simulink model "Copy_of_AB_Final_of_MPC_Bandwidth_Result"  (R2022b)
settings: Solver=FixedStepDiscrete  StartTime=0.0  StopTime=Inf  FixedStep=100e-6  RelTol=1e-3  EnableMultiTasking=on
undefined symbols (not defined in the file): C28x, CPU1, CPU2, CurrentBypassValue, DiscIntNeverNeededParam, Down, GPTRIP1SEL, TZ1, Up
libraries: c2802xlib x31, simulink x22, dspstat3 x17, dspsigops x9, c2837xDlib x6, c280xlib x5, PID_Lib x2, c2000lib x1, spsAlphaBetaZerotoabcLib x1, spsAlphaBetaZerotodq0Lib x1
(part 8 of 8)

== system Copy_of_AB_Final_of_MPC_Bandwidth_Result/Subsystem1/GridCurrentSecondPrediction/CostFunctionofVoltageVectors/CostFunctionVoltage3/QGridCurrentSecondPrediction_Voltage3 ==
  MPCC_f32Predictionterm_A : Inport
  MPCC_f32Predictionterm_B : Inport  Port=2
  MPCC_f32Predictionterm_C : Inport  Port=3
  MPCC_f32DGridCurrent_K_1 : Inport  Port=4
  MPCC_f32QGridCurrent_K_1 : Inport  Port=5
  MPCC_f32QGridVoltage : Inport  Port=6
  MPCC_f32QVoltageVector3 : Inport  Port=7
  Add1 : Sum  Inputs=+-+-
  Gain : Gain  Gain=0
  Product : Product
  Product1 : Product
  Product2 : Product  OutDataTypeStr=Inherit: Inherit via back propagation
  Product4 : Product
  MPCC_f32QGridCurrent_K_2_Voltage3 : Outport
  wires:
  [MPCC_f32QGridCurrent_K_1] -> Product/2
  MPCC_f32Predictionterm_A/1 -> [MPCC_f32Predictionterm_A]
  [MPCC_f32QGridVoltage] -> Product2/2
  Product1/1 -> Gain/1
  [MPCC_f32Predictionterm_C] -> Product1/1
  Product/1 -> Add1/1
  [MPCC_f32QVoltageVector3] -> Product4/2
  [MPCC_f32Predictionterm_A] -> Product/1
  [MPCC_f32Predictionterm_B] -> Product4/1
  [MPCC_f32Predictionterm_B] -> Product2/1
  [MPCC_f32DGridCurrent_K_1] -> Product1/2
  MPCC_f32DGridCurrent_K_1/1 -> [MPCC_f32DGridCurrent_K_1]
  MPCC_f32QGridCurrent_K_1/1 -> [MPCC_f32QGridCurrent_K_1]
  MPCC_f32Predictionterm_C/1 -> [MPCC_f32Predictionterm_C]
  MPCC_f32QGridVoltage/1 -> [MPCC_f32QGridVoltage]
  MPCC_f32Predictionterm_B/1 -> [MPCC_f32Predictionterm_B]
  Add1/1 -> MPCC_f32QGridCurrent_K_2_Voltage3/1
  MPCC_f32QVoltageVector3/1 -> [MPCC_f32QVoltageVector3]
  Product2/1 -> Add1/3
  Product4/1 -> Add1/4
  Gain/1 -> Add1/2

== system Copy_of_AB_Final_of_MPC_Bandwidth_Result/Subsystem1/GridCurrentSecondPrediction/CostFunctionofVoltageVectors/CostFunctionVoltage4/CostFunctionVoltage4 ==
  MPCC_f32DGridCurrentReference : Inport
  MPCC_f32QGridCurrentReference : Inport  Port=2
  MPCC_f32DGridCurrent_K_2_Voltage4 : Inport  Port=3
  MPCC_f32QGridCurrent_K_2_Voltage4 : Inport  Port=4
  MPCC_f32DGridCurrent : Inport  Port=5
  MPCC_f32QGridCurrent : Inport  Port=6
  MPCC_f32DGridCurrent1 : Inport  Port=7
  MPCC_f32QGridCurrent1 : Inport  Port=8
  Abs{,1..5} (6 alike) : Abs  SaturateOnIntegerOverflow=off
  Add{,2..6} (6 alike) : Sum  Inputs=+-
  Add1 : Sum  Inputs=++++++
  Constant : Constant  Value=single(0)
  Constant1 : Constant  Value=single(0)
  Gain : Gain
  Gain1 : Gain
  Gain2 : Gain  Gain=0
  Gain3 : Gain  Gain=0
  Square : Math  Operator=square
  Square1 : Math  Operator=square
  MPCC_f32CostFunction_Voltage4 : Outport
  wires:
  MPCC_f32QGridCurrentReference/1 -> [MPCC_f32QGridCurrentReference]
  MPCC_f32DGridCurrentReference/1 -> [MPCC_f32DGridCurrentReference]
  MPCC_f32QGridCurrent_K_2_Voltage4/1 -> [MPCC_f32QGridCurrent_K_2_Voltage4]
  MPCC_f32DGridCurrent_K_2_Voltage4/1 -> [MPCC_f32DGridCurrent_K_2_Voltage4]
  [MPCC_f32DGridCurrentReference] -> Add/1
  [MPCC_f32DGridCurrent_K_2_Voltage4] -> Add/2
  [MPCC_f32QGridCurrentReference] -> Add2/1
  [MPCC_f32QGridCurrent_K_2_Voltage4] -> Add2/2
  MPCC_f32QGridCurrent/1 -> [MPCC_f32QGridCurrent]
  MPCC_f32DGridCurrent/1 -> [MPCC_f32DGridCurrent]
  [MPCC_f32QGridCurrent] -> Add4/1
  Add4/1 -> Abs3/1
  Add3/1 -> Abs2/1
  [MPCC_f32QGridCurrent_K_2_Voltage4] -> Add4/2
  [MPCC_f32DGridCurrent] -> Add3/1
  [MPCC_f32DGridCurrent_K_2_Voltage4] -> Add3/2
  Abs2/1 -> Gain/1
  Abs3/1 -> Gain1/1
  Add1/1 -> MPCC_f32CostFunction_Voltage4/1
  Gain/1 -> Add1/3
  Gain1/1 -> Add1/4
  Abs1/1 -> Add1/2
  Add2/1 -> Abs1/1
  Abs/1 -> Add1/1
  Add/1 -> Abs/1
  MPCC_f32DGridCurrent1/1 -> [MPCC_f32DGridCurrent1]
  MPCC_f32QGridCurrent1/1 -> [MPCC_f32QGridCurrent1]
  Constant/1 -> Add5/1
  Add5/1 -> Abs4/1
  Add6/1 -> Abs5/1
  Abs4/1 -> Gain2/1
  Constant1/1 -> Add6/1
  [MPCC_f32DGridCurrent1] -> Add6/2
  [MPCC_f32QGridCurrent1] -> Add5/2
  Gain2/1 -> Add1/6
  Abs5/1 -> Gain3/1
  Gain3/1 -> Add1/5

== system Copy_of_AB_Final_of_MPC_Bandwidth_Result/Subsystem1/GridCurrentSecondPrediction/CostFunctionofVoltageVectors/CostFunctionVoltage4/DGridCurrentSecondPrediction_Voltage4 ==
  MPCC_f32Predictionterm_A : Inport
  MPCC_f32Predictionterm_B : Inport  Port=2
  MPCC_f32Predictionterm_C : Inport  Port=3
  MPCC_f32DGridCurrent_K_1 : Inport  Port=4
  MPCC_f32QGridCurrent_K_1 : Inport  Port=5
  MPCC_f32DGridVoltage : Inport  Port=6
  MPCC_f32DVoltageVector4 : Inport  Port=7
  Add1 : Sum  Inputs=+++-
  Gain : Gain  Gain=0
  Product : Product
  Product1 : Product
  Product2 : Product  OutDataTypeStr=Inherit: Inherit via back propagation
  Product4 : Product
  MPCC_f32DGridCurrent_K_2_Voltage4 : Outport
  wires:
  [MPCC_f32DGridCurrent_K_1] -> Product/2
  MPCC_f32Predictionterm_A/1 -> [MPCC_f32Predictionterm_A]
  [MPCC_f32DGridVoltage] -> Product2/2
  Product1/1 -> Gain/1
  [MPCC_f32Predictionterm_C] -> Product1/1
  Product/1 -> Add1/1
  [MPCC_f32DVoltageVector4] -> Product4/2
  MPCC_f32DGridVoltage/1 -> [MPCC_f32DGridVoltage]
  [MPCC_f32Predictionterm_A] -> Product/1
  [MPCC_f32Predictionterm_B] -> Product4/1
  [MPCC_f32Predictionterm_B] -> Product2/1
  [MPCC_f32QGridCurrent_K_1] -> Product1/2
  MPCC_f32DGridCurrent_K_1/1 -> [MPCC_f32DGridCurrent_K_1]
  MPCC_f32QGridCurrent_K_1/1 -> [MPCC_f32QGridCurrent_K_1]
  MPCC_f32Predictionterm_C/1 -> [MPCC_f32Predictionterm_C]
  MPCC_f32Predictionterm_B/1 -> [MPCC_f32Predictionterm_B]
  Add1/1 -> MPCC_f32DGridCurrent_K_2_Voltage4/1
  MPCC_f32DVoltageVector4/1 -> [MPCC_f32DVoltageVector4]
  Product2/1 -> Add1/3
  Product4/1 -> Add1/4
  Gain/1 -> Add1/2

== system Copy_of_AB_Final_of_MPC_Bandwidth_Result/Subsystem1/GridCurrentSecondPrediction/CostFunctionofVoltageVectors/CostFunctionVoltage4/QGridCurrentSecondPrediction_Voltage4 ==
  MPCC_f32Predictionterm_A : Inport
  MPCC_f32Predictionterm_B : Inport  Port=2
  MPCC_f32Predictionterm_C : Inport  Port=3
  MPCC_f32DGridCurrent_K_1 : Inport  Port=4
  MPCC_f32QGridCurrent_K_1 : Inport  Port=5
  MPCC_f32QGridVoltage : Inport  Port=6
  MPCC_f32QVoltageVector4 : Inport  Port=7
  Add1 : Sum  Inputs=+-+-
  Gain : Gain  Gain=0
  Product : Product
  Product1 : Product
  Product2 : Product  OutDataTypeStr=Inherit: Inherit via back propagation
  Product4 : Product  OutDataTypeStr=Inherit: Inherit via back propagation
  MPCC_f32QGridCurrent_K_2_Voltage4 : Outport
  wires:
  [MPCC_f32QGridCurrent_K_1] -> Product/2
  MPCC_f32Predictionterm_A/1 -> [MPCC_f32Predictionterm_A]
  [MPCC_f32QGridVoltage] -> Product2/2
  Product1/1 -> Gain/1
  [MPCC_f32Predictionterm_C] -> Product1/1
  Product/1 -> Add1/1
  [MPCC_f32QVoltageVector4] -> Product4/2
  [MPCC_f32Predictionterm_A] -> Product/1
  [MPCC_f32Predictionterm_B] -> Product4/1
  [MPCC_f32Predictionterm_B] -> Product2/1
  [MPCC_f32DGridCurrent_K_1] -> Product1/2
  MPCC_f32DGridCurrent_K_1/1 -> [MPCC_f32DGridCurrent_K_1]
  MPCC_f32QGridCurrent_K_1/1 -> [MPCC_f32QGridCurrent_K_1]
  MPCC_f32Predictionterm_C/1 -> [MPCC_f32Predictionterm_C]
  MPCC_f32QGridVoltage/1 -> [MPCC_f32QGridVoltage]
  MPCC_f32Predictionterm_B/1 -> [MPCC_f32Predictionterm_B]
  Add1/1 -> MPCC_f32QGridCurrent_K_2_Voltage4/1
  MPCC_f32QVoltageVector4/1 -> [MPCC_f32QVoltageVector4]
  Product2/1 -> Add1/3
  Product4/1 -> Add1/4
  Gain/1 -> Add1/2

== system Copy_of_AB_Final_of_MPC_Bandwidth_Result/Subsystem1/GridCurrentSecondPrediction/CostFunctionofVoltageVectors/CostFunctionVoltage5/CostFunctionVoltage5 ==
  MPCC_f32DGridCurrentReference : Inport
  MPCC_f32QGridCurrentReference : Inport  Port=2
  MPCC_f32DGridCurrent_K_2_Voltage5 : Inport  Port=3
  MPCC_f32QGridCurrent_K_2_Voltage5 : Inport  Port=4
  MPCC_f32DGridCurrent : Inport  Port=5
  MPCC_f32QGridCurrent : Inport  Port=6
  MPCC_f32DGridCurrent1 : Inport  Port=7
  MPCC_f32QGridCurrent1 : Inport  Port=8
  Abs{,1..5} (6 alike) : Abs  SaturateOnIntegerOverflow=off
  Add{,2..6} (6 alike) : Sum  Inputs=+-
  Add1 : Sum  Inputs=++++++
  Constant : Constant  Value=single(0)
  Constant1 : Constant  Value=single(0)
  Gain : Gain
  Gain1 : Gain
  Gain2 : Gain  Gain=0
  Gain3 : Gain  Gain=0
  Square : Math  Operator=square
  Square1 : Math  Operator=square
  MPCC_f32CostFunction_Voltage5 : Outport
  wires:
  MPCC_f32QGridCurrentReference/1 -> [MPCC_f32QGridCurrentReference]
  MPCC_f32DGridCurrentReference/1 -> [MPCC_f32DGridCurrentReference]
  MPCC_f32QGridCurrent_K_2_Voltage5/1 -> [MPCC_f32QGridCurrent_K_2_Voltage5]
  MPCC_f32DGridCurrent_K_2_Voltage5/1 -> [MPCC_f32DGridCurrent_K_2_Voltage5]
  [MPCC_f32DGridCurrentReference] -> Add/1
  [MPCC_f32DGridCurrent_K_2_Voltage5] -> Add/2
  [MPCC_f32QGridCurrentReference] -> Add2/1
  [MPCC_f32QGridCurrent_K_2_Voltage5] -> Add2/2
  MPCC_f32QGridCurrent/1 -> [MPCC_f32QGridCurrent]
  MPCC_f32DGridCurrent/1 -> [MPCC_f32DGridCurrent]
  [MPCC_f32QGridCurrent] -> Add4/1
  Add4/1 -> Abs3/1
  Add3/1 -> Abs2/1
  [MPCC_f32QGridCurrent_K_2_Voltage5] -> Add4/2
  [MPCC_f32DGridCurrent] -> Add3/1
  [MPCC_f32DGridCurrent_K_2_Voltage5] -> Add3/2
  Abs2/1 -> Gain/1
  Abs3/1 -> Gain1/1
  Add1/1 -> MPCC_f32CostFunction_Voltage5/1
  Gain/1 -> Add1/3
  Gain1/1 -> Add1/4
  Abs1/1 -> Add1/2
  Add2/1 -> Abs1/1
  Abs/1 -> Add1/1
  Add/1 -> Abs/1
  MPCC_f32DGridCurrent1/1 -> [MPCC_f32DGridCurrent1]
  MPCC_f32QGridCurrent1/1 -> [MPCC_f32QGridCurrent1]
  Constant/1 -> Add5/1
  Add5/1 -> Abs4/1
  Add6/1 -> Abs5/1
  Abs4/1 -> Gain2/1
  Constant1/1 -> Add6/1
  [MPCC_f32DGridCurrent1] -> Add6/2
  [MPCC_f32QGridCurrent1] -> Add5/2
  Gain2/1 -> Add1/6
  Abs5/1 -> Gain3/1
  Gain3/1 -> Add1/5

== system Copy_of_AB_Final_of_MPC_Bandwidth_Result/Subsystem1/GridCurrentSecondPrediction/CostFunctionofVoltageVectors/CostFunctionVoltage5/DGridCurrentSecondPrediction_Voltage5 ==
  MPCC_f32Predictionterm_A : Inport
  MPCC_f32Predictionterm_B : Inport  Port=2
  MPCC_f32Predictionterm_C : Inport  Port=3
  MPCC_f32DGridCurrent_K_1 : Inport  Port=4
  MPCC_f32QGridCurrent_K_1 : Inport  Port=5
  MPCC_f32DGridVoltage : Inport  Port=6
  MPCC_f32DVoltageVector5 : Inport  Port=7
  Add1 : Sum  Inputs=+++-
  Gain : Gain  Gain=0
  Product : Product
  Product1 : Product
  Product2 : Product  OutDataTypeStr=Inherit: Inherit via back propagation
  Product4 : Product
  MPCC_f32DGridCurrent_K_2_Voltage5 : Outport
  wires:
  [MPCC_f32DGridCurrent_K_1] -> Product/2
  MPCC_f32Predictionterm_A/1 -> [MPCC_f32Predictionterm_A]
  [MPCC_f32DGridVoltage] -> Product2/2
  Product1/1 -> Gain/1
  [MPCC_f32Predictionterm_C] -> Product1/1
  Product/1 -> Add1/1
  [MPCC_f32DVoltageVector5] -> Product4/2
  MPCC_f32DGridVoltage/1 -> [MPCC_f32DGridVoltage]
  [MPCC_f32Predictionterm_A] -> Product/1
  [MPCC_f32Predictionterm_B] -> Product4/1
  [MPCC_f32Predictionterm_B] -> Product2/1
  [MPCC_f32QGridCurrent_K_1] -> Product1/2
  MPCC_f32DGridCurrent_K_1/1 -> [MPCC_f32DGridCurrent_K_1]
  MPCC_f32QGridCurrent_K_1/1 -> [MPCC_f32QGridCurrent_K_1]
  MPCC_f32Predictionterm_C/1 -> [MPCC_f32Predictionterm_C]
  MPCC_f32Predictionterm_B/1 -> [MPCC_f32Predictionterm_B]
  Add1/1 -> MPCC_f32DGridCurrent_K_2_Voltage5/1
  MPCC_f32DVoltageVector5/1 -> [MPCC_f32DVoltageVector5]
  Product2/1 -> Add1/3
  Product4/1 -> Add1/4
  Gain/1 -> Add1/2

== system Copy_of_AB_Final_of_MPC_Bandwidth_Result/Subsystem1/GridCurrentSecondPrediction/CostFunctionofVoltageVectors/CostFunctionVoltage5/QGridCurrentSecondPrediction_Voltage5 ==
  MPCC_f32Predictionterm_A : Inport
  MPCC_f32Predictionterm_B : Inport  Port=2
  MPCC_f32Predictionterm_C : Inport  Port=3
  MPCC_f32DGridCurrent_K_1 : Inport  Port=4
  MPCC_f32QGridCurrent_K_1 : Inport  Port=5
  MPCC_f32QGridVoltage : Inport  Port=6
  MPCC_f32QVoltageVector5 : Inport  Port=7
  Add1 : Sum  Inputs=+-+-
  Gain : Gain  Gain=0
  Product : Product
  Product1 : Product
  Product2 : Product  OutDataTypeStr=Inherit: Inherit via back propagation
  Product4 : Product
  MPCC_f32QGridCurrent_K_2_Voltage5 : Outport
  wires:
  [MPCC_f32QGridCurrent_K_1] -> Product/2
  MPCC_f32Predictionterm_A/1 -> [MPCC_f32Predictionterm_A]
  [MPCC_f32QGridVoltage] -> Product2/2
  Product1/1 -> Gain/1
  [MPCC_f32Predictionterm_C] -> Product1/1
  Product/1 -> Add1/1
  [MPCC_f32QVoltageVector5] -> Product4/2
  [MPCC_f32Predictionterm_A] -> Product/1
  [MPCC_f32Predictionterm_B] -> Product4/1
  [MPCC_f32Predictionterm_B] -> Product2/1
  [MPCC_f32DGridCurrent_K_1] -> Product1/2
  MPCC_f32DGridCurrent_K_1/1 -> [MPCC_f32DGridCurrent_K_1]
  MPCC_f32QGridCurrent_K_1/1 -> [MPCC_f32QGridCurrent_K_1]
  MPCC_f32Predictionterm_C/1 -> [MPCC_f32Predictionterm_C]
  MPCC_f32QGridVoltage/1 -> [MPCC_f32QGridVoltage]
  MPCC_f32Predictionterm_B/1 -> [MPCC_f32Predictionterm_B]
  Add1/1 -> MPCC_f32QGridCurrent_K_2_Voltage5/1
  MPCC_f32QVoltageVector5/1 -> [MPCC_f32QVoltageVector5]
  Product2/1 -> Add1/3
  Product4/1 -> Add1/4
  Gain/1 -> Add1/2

== system Copy_of_AB_Final_of_MPC_Bandwidth_Result/Subsystem1/GridCurrentSecondPrediction/CostFunctionofVoltageVectors/CostFunctionVoltage6/CostFunctionVoltage6 ==
  MPCC_f32DGridCurrentReference : Inport
  MPCC_f32QGridCurrentReference : Inport  Port=2
  MPCC_f32DGridCurrent_K_2_Voltage6 : Inport  Port=3
  MPCC_f32QGridCurrent_K_2_Voltage6 : Inport  Port=4
  MPCC_f32DGridCurrent : Inport  Port=5
  MPCC_f32QGridCurrent : Inport  Port=6
  MPCC_f32DGridCurrent1 : Inport  Port=7
  MPCC_f32QGridCurrent1 : Inport  Port=8
  Abs{,1..5} (6 alike) : Abs  SaturateOnIntegerOverflow=off
  Add{,2..6} (6 alike) : Sum  Inputs=+-
  Add1 : Sum  Inputs=++++++
  Constant : Constant  Value=single(0)
  Constant1 : Constant  Value=single(0)
  Gain : Gain
  Gain1 : Gain
  Gain2 : Gain  Gain=0
  Gain3 : Gain  Gain=0
  Square : Math  Operator=square
  Square1 : Math  Operator=square
  MPCC_f32CostFunction_Voltage6 : Outport
  wires:
  MPCC_f32QGridCurrentReference/1 -> [MPCC_f32QGridCurrentReference]
  MPCC_f32DGridCurrentReference/1 -> [MPCC_f32DGridCurrentReference]
  MPCC_f32QGridCurrent_K_2_Voltage6/1 -> [MPCC_f32QGridCurrent_K_2_Voltage6]
  MPCC_f32DGridCurrent_K_2_Voltage6/1 -> [MPCC_f32DGridCurrent_K_2_Voltage6]
  [MPCC_f32DGridCurrentReference] -> Add/1
  [MPCC_f32DGridCurrent_K_2_Voltage6] -> Add/2
  [MPCC_f32QGridCurrentReference] -> Add2/1
  [MPCC_f32QGridCurrent_K_2_Voltage6] -> Add2/2
  MPCC_f32QGridCurrent/1 -> [MPCC_f32QGridCurrent]
  MPCC_f32DGridCurrent/1 -> [MPCC_f32DGridCurrent]
  [MPCC_f32QGridCurrent] -> Add4/1
  Add4/1 -> Abs3/1
  Add3/1 -> Abs2/1
  [MPCC_f32QGridCurrent_K_2_Voltage6] -> Add4/2
  [MPCC_f32DGridCurrent] -> Add3/1
  [MPCC_f32DGridCurrent_K_2_Voltage6] -> Add3/2
  Abs2/1 -> Gain/1
  Abs3/1 -> Gain1/1
  Add1/1 -> MPCC_f32CostFunction_Voltage6/1
  Gain/1 -> Add1/3
  Gain1/1 -> Add1/4
  Abs1/1 -> Add1/2
  Add2/1 -> Abs1/1
  Abs/1 -> Add1/1
  Add/1 -> Abs/1
  MPCC_f32DGridCurrent1/1 -> [MPCC_f32DGridCurrent1]
  MPCC_f32QGridCurrent1/1 -> [MPCC_f32QGridCurrent1]
  Constant/1 -> Add5/1
  Add5/1 -> Abs4/1
  Add6/1 -> Abs5/1
  Abs4/1 -> Gain2/1
  Constant1/1 -> Add6/1
  [MPCC_f32DGridCurrent1] -> Add6/2
  [MPCC_f32QGridCurrent1] -> Add5/2
  Gain2/1 -> Add1/6
  Abs5/1 -> Gain3/1
  Gain3/1 -> Add1/5

== system Copy_of_AB_Final_of_MPC_Bandwidth_Result/Subsystem1/GridCurrentSecondPrediction/CostFunctionofVoltageVectors/CostFunctionVoltage6/DGridCurrentSecondPrediction_Voltage6 ==
  MPCC_f32Predictionterm_A : Inport
  MPCC_f32Predictionterm_B : Inport  Port=2
  MPCC_f32Predictionterm_C : Inport  Port=3
  MPCC_f32DGridCurrent_K_1 : Inport  Port=4
  MPCC_f32QGridCurrent_K_1 : Inport  Port=5
  MPCC_f32DGridVoltage : Inport  Port=6
  MPCC_f32DVoltageVector6 : Inport  Port=7
  Add1 : Sum  Inputs=+++-
  Gain : Gain  Gain=0
  Product : Product
  Product1 : Product
  Product2 : Product  OutDataTypeStr=Inherit: Inherit via back propagation
  Product4 : Product
  MPCC_f32DGridCurrent_K_2_Voltage6 : Outport
  wires:
  [MPCC_f32DGridCurrent_K_1] -> Product/2
  MPCC_f32Predictionterm_A/1 -> [MPCC_f32Predictionterm_A]
  [MPCC_f32DGridVoltage] -> Product2/2
  Product1/1 -> Gain/1
  [MPCC_f32Predictionterm_C] -> Product1/1
  Product/1 -> Add1/1
  [MPCC_f32DVoltageVector6] -> Product4/2
  MPCC_f32DGridVoltage/1 -> [MPCC_f32DGridVoltage]
  [MPCC_f32Predictionterm_A] -> Product/1
  [MPCC_f32Predictionterm_B] -> Product4/1
  [MPCC_f32Predictionterm_B] -> Product2/1
  [MPCC_f32QGridCurrent_K_1] -> Product1/2
  MPCC_f32DGridCurrent_K_1/1 -> [MPCC_f32DGridCurrent_K_1]
  MPCC_f32QGridCurrent_K_1/1 -> [MPCC_f32QGridCurrent_K_1]
  MPCC_f32Predictionterm_C/1 -> [MPCC_f32Predictionterm_C]
  MPCC_f32Predictionterm_B/1 -> [MPCC_f32Predictionterm_B]
  Add1/1 -> MPCC_f32DGridCurrent_K_2_Voltage6/1
  MPCC_f32DVoltageVector6/1 -> [MPCC_f32DVoltageVector6]
  Product2/1 -> Add1/3
  Product4/1 -> Add1/4
  Gain/1 -> Add1/2

== system Copy_of_AB_Final_of_MPC_Bandwidth_Result/Subsystem1/GridCurrentSecondPrediction/CostFunctionofVoltageVectors/CostFunctionVoltage6/QGridCurrentSecondPrediction_Voltage6 ==
  MPCC_f32Predictionterm_A : Inport
  MPCC_f32Predictionterm_B : Inport  Port=2
  MPCC_f32Predictionterm_C : Inport  Port=3
  MPCC_f32DGridCurrent_K_1 : Inport  Port=4
  MPCC_f32QGridCurrent_K_1 : Inport  Port=5
  MPCC_f32QGridVoltage : Inport  Port=6
  MPCC_f32QVoltageVector6 : Inport  Port=7
  Add1 : Sum  Inputs=+-+-
  Gain : Gain  Gain=0
  Product : Product
  Product1 : Product
  Product2 : Product  OutDataTypeStr=Inherit: Inherit via back propagation
  Product4 : Product
  MPCC_f32QGridCurrent_K_2_Voltage6 : Outport
  wires:
  [MPCC_f32QGridCurrent_K_1] -> Product/2
  MPCC_f32Predictionterm_A/1 -> [MPCC_f32Predictionterm_A]
  [MPCC_f32QGridVoltage] -> Product2/2
  Product1/1 -> Gain/1
  [MPCC_f32Predictionterm_C] -> Product1/1
  Product/1 -> Add1/1
  [MPCC_f32QVoltageVector6] -> Product4/2
  [MPCC_f32Predictionterm_A] -> Product/1
  [MPCC_f32Predictionterm_B] -> Product4/1
  [MPCC_f32Predictionterm_B] -> Product2/1
  [MPCC_f32DGridCurrent_K_1] -> Product1/2
  MPCC_f32DGridCurrent_K_1/1 -> [MPCC_f32DGridCurrent_K_1]
  MPCC_f32QGridCurrent_K_1/1 -> [MPCC_f32QGridCurrent_K_1]
  MPCC_f32Predictionterm_C/1 -> [MPCC_f32Predictionterm_C]
  MPCC_f32QGridVoltage/1 -> [MPCC_f32QGridVoltage]
  MPCC_f32Predictionterm_B/1 -> [MPCC_f32Predictionterm_B]
  Add1/1 -> MPCC_f32QGridCurrent_K_2_Voltage6/1
  MPCC_f32QVoltageVector6/1 -> [MPCC_f32QVoltageVector6]
  Product2/1 -> Add1/3
  Product4/1 -> Add1/4
  Gain/1 -> Add1/2

== stateflow chart Copy_of_AB_Final_of_MPC_Bandwidth_Result/Chart1 ==
  state GPin_FC [parallel]
    settings: executionOrder=1
    state Rate_100us
      on every(1,tic): send(GPin_FC);
    (default) -> GPin_FC.Rate_100us : /{send(GPin_FC);}
  state ADC_FC [parallel]
    settings: executionOrder=2
    state Rate_100us
      on every(1,tic): send(ADC_FC);
    (default) -> ADC_FC.Rate_100us : /{send(ADC_FC);}
  state PLL_FC [parallel]
    settings: executionOrder=3
    state Rate_100us
      on every(1,tic): send(PLL_FC);
    (default) -> PLL_FC.Rate_100us : /{send(PLL_FC);}
  state CurrentLoop_FC [parallel]
    settings: executionOrder=4
    state Rate_100us
      on every(1,tic): send(CurrentLoop_FC);
    (default) -> CurrentLoop_FC.Rate_100us : /{send(CurrentLoop_FC);}
  state VoltageLoop_FC [parallel]
    settings: executionOrder=5
    state Rate_1000us
      on every(10,tic): send(VoltageLoop_FC);
    (default) -> Rate_1000us : /{send(VoltageLoop_FC);}
  state GPout_FC [parallel]
    settings: executionOrder=6
    state Rate_100us
      on every(1,tic): send(GPout_FC);
    (default) -> GPout_FC.Rate_100us : /{send(GPout_FC);}
  events: ADC_FC output FUNCTION_CALL_EVENT; PLL_FC output FUNCTION_CALL_EVENT; tic input FUNCTION_CALL_EVENT; CurrentLoop_FC output FUNCTION_CALL_EVENT; VoltageLoop_FC output FUNCTION_CALL_EVENT; GPin_FC output FUNCTION_CALL_EVENT; GPout_FC output FUNCTION_CALL_EVENT
